simulink model "BATTERYMANAGEMENTSYSTEM"  (R2023b)
settings: Solver=VariableStepAuto  StartTime=0.0  StopTime=10.0  RelTol=1e-3
settings Model: Creator=lucaerviati  LastModifiedBy=carol
settings OptimizationCC: ReuseModelBlockBuffer=off

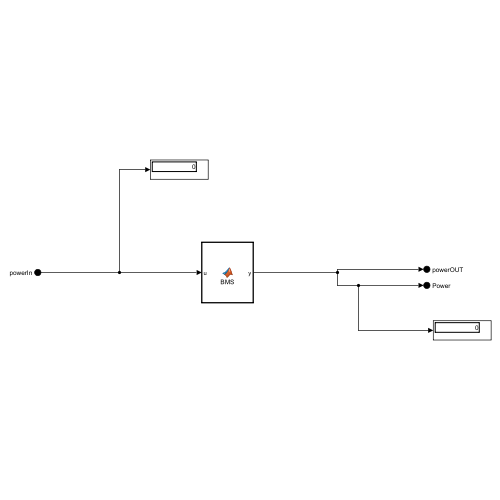
[thumbnail: Simulink's stored preview of the top-level diagram]
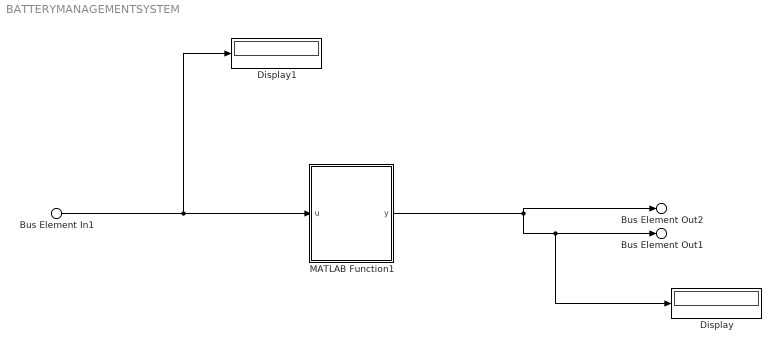
== system BATTERYMANAGEMENTSYSTEM ==
  Bus Element In1 : Inport  PortName=powerIn
  Display : Display
  Display1 : Display
  MATLAB Function1 : MATLAB Function  TreatAsAtomicUnit=on
  Bus Element Out2 : Outport  PortName=powerOUT
  Bus Element Out1 : Outport  Port=2  PortName=Power
  wires:
  MATLAB Function1/1(y) -> Bus Element Out2/1, Bus Element Out1/1, Display/1
  Bus Element In1/1 -> Display1/1, MATLAB Function1/1(u)

== matlab function BATTERYMANAGEMENTSYSTEM/MATLAB Function1 ==
  data: u input; y output
function y = BMS(u)


if u<12
    y = 0;
elseif u>12
    y = 0;    
else
    y = 12;
end




y = u;
